simulink model "DC_motor_vel"  (R2018b)
settings: Solver=VariableStepAuto  StartTime=0.0  StopTime=12  RelTol=1e-3
settings Model: Creator=EMiR  LastModifiedBy=EMiR

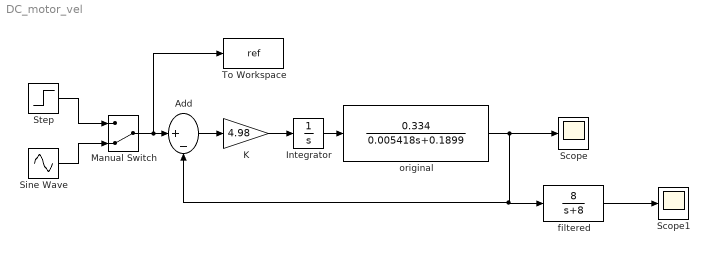
== system DC_motor_vel ==
  Add : Sum  Inputs=|+-
  Integrator : Integrator
  K : Gain  Gain=4.98
  Manual Switch : ManualSwitch  CurrentSetting=0
  Scope : Scope
  Scope1 : Scope
  Sine Wave : Sin  Amplitude=11  SampleTime=0
  Step : Step  After=11  SampleTime=0
  To Workspace : ToWorkspace  VariableName=ref  SampleTime=-1
  filtered : TransferFcn  Numerator=[8]  Denominator=[1 8]
  original : TransferFcn  Numerator=[0.334]  Denominator=[0.005418 0.1899]
  wires:
  Step/1 -> Manual Switch/1
  Sine Wave/1 -> Manual Switch/2
  Manual Switch/1 -> To Workspace/1, Add/1
  Add/1 -> K/1
  K/1 -> Integrator/1
  Integrator/1 -> original/1
  original/1 -> filtered/1, Add/2, Scope/1
  filtered/1 -> Scope1/1
